simulink model "simulace_zar"  (R2022b)
settings: Solver=VariableStepAuto  StartTime=0.0  StopTime=10.0  RelTol=1e-3
settings Model: Creator=honza  LastModifiedBy=honza

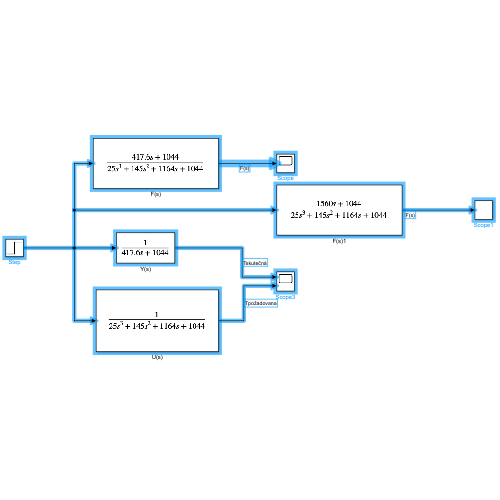
[thumbnail: Simulink's stored preview of the top-level diagram]
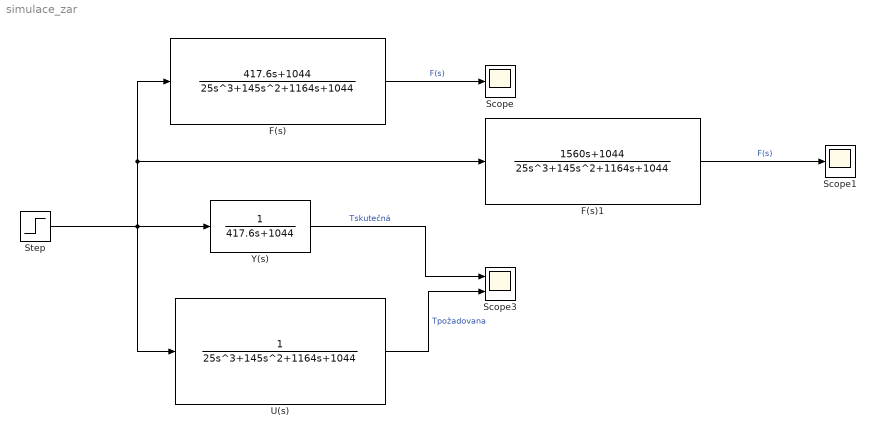
== system simulace_zar ==
  F(s) : TransferFcn  Numerator=[417.6 1044]  Denominator=[25 145 1164 1044]
  F(s)1 : TransferFcn  Numerator=[1560 1044]  Denominator=[25 145 1164 1044]
  Scope : Scope
  Scope1 : Scope
  Scope3 : Scope  NumInputPorts=2
  Step : Step  Time=0  After=200  SampleTime=0
  U(s) : TransferFcn  Denominator=[25 145 1164 1044]
  Y(s) : TransferFcn  Denominator=[417.6 1044]
  wires:
  F(s)1/1 -> Scope1/1  "F(s)"
  U(s)/1 -> Scope3/2  "Tpožadovana"
  Step/1 -> F(s)1/1, F(s)/1, Y(s)/1, U(s)/1
  Y(s)/1 -> Scope3/1  "Tskutečná"
  F(s)/1 -> Scope/1  "F(s)"
